simulink model "week2_problem4"  (R2019b)
settings: Solver=VariableStepAuto  StartTime=0.0  StopTime=10.0  RelTol=1e-3
model workspace (MAT data in the model file):
  J = 3.2284e-06
  Ke = 0.0274
  Kt = 0.0274
  L = 2.75e-06
  R = 4
  b = 3.5077e-06
settings Model: Creator=Shreyas  LastModifiedBy=Shreyas

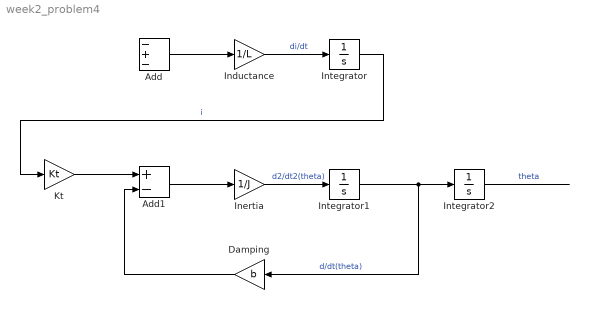
== system week2_problem4 ==
  Add : Sum  Inputs=-+-
  Add1 : Sum  Inputs=+-
  Damping : Gain  Gain=b
  Inductance : Gain  Gain=1/L
  Inertia : Gain  Gain=1/J
  Integrator : Integrator
  Integrator1 : Integrator
  Integrator2 : Integrator
  Kt : Gain  Gain=Kt
  wires:
  Integrator1/1 -> Damping/1, Integrator2/1  "d/dt(theta)"
  Inductance/1 -> Integrator/1  "di/dt"
  Integrator/1 -> Kt/1  "i"
  Inertia/1 -> Integrator1/1  "d2/dt2(theta)"
  Integrator2/1 -> ?  "theta"
  Add/1 -> Inductance/1
  Add1/1 -> Inertia/1
  Kt/1 -> Add1/1
  Damping/1 -> Add1/2
